simulink model "test_velocity_control_2"  (R2015a)
settings: Solver=FixedStepDiscrete  StartTime=0.0  StopTime=inf  FixedStep=sample_time  RelTol=1e-3
undefined symbols (not defined in the file or in its folder): A_lpf_fourbar_angles, A_lpf_imu, A_lpf_lateral_angle, B1_lpf_fourbar_angles, B1_lpf_imu, B1_lpf_lateral_angle, B2_lpf_fourbar_angles, B2_lpf_imu, B2_lpf_lateral_angle, control_start_time, kp_velocity_swing_trajectory, sample_time, swing_test_frequency, swing_test_leg_angle_amplitude, swing_test_leg_angle_bias, swing_test_leg_length_amplitude, swing_test_leg_length_bias, swing_test_length_angle_phase, swing_test_right_left_phase
libraries: simulink x6
settings Model: CovSFcnEnable=off  Creator=wmartin  LastModifiedBy=wmartin
settings SolverCC: EnableConcurrentExecution=on
settings DataIOCC: LimitDataPoints=off  MaxDataPoints=1000000000  SaveFormat=StructureWithTime  SignalLogging=off  DSMLogging=off  VisualizeSimOutput=off
settings OptimizationCC: BlockReduction=off  OptimizeBlockIOStorage=off  BufferReuse=off  GlobalBufferReuse=off  ExpressionFolding=off  ExpressionDepthLimit=2147483647  LocalBlockOutputs=off  SimCompilerOptimization=on
settings DebuggingCC: UnderspecifiedInitializationDetection=Classic  MergeDetectMultiDrivingBlocksExec=none  SolverPrmCheckMsg=warning  StateNameClashWarn=warning
settings HardwareCC: ProdIntDivRoundTo=Zero  ProdEndianess=LittleEndian  ProdLongLongMode=on  ProdHWDeviceType=Generic->32-bit x86 compatible
settings ModelReferenceCC: UpdateModelReferenceTargets=IfOutOfDate  ModelReferenceNumInstancesAllowed=Single  ModelReferenceMinAlgLoopOccurrences=on
settings RTWCC: SystemTargetFile=slrt.tlc  TemplateMakefile=slrt_default_tmf  Description=Simulink Real-Time  RTWVerbose=off  RTWCompilerOptimization=on
settings CodeAppCC: MaxIdLength=256
settings SimulinkRealTimeCC: GeneratePreprocessorConditionals=Disable all  RL32LogBufSizeModifier=1e8

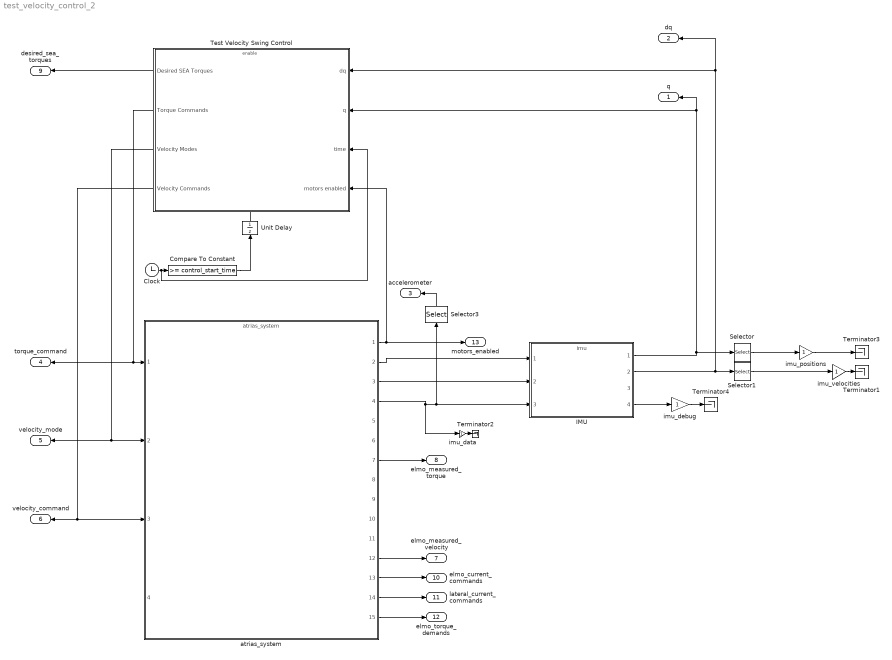
== system test_velocity_control_2 ==
  Clock : Clock
  Compare To Constant : simulink/Logic and Bit Operations/Compare To Constant  relop=>=  const=control_start_time  OutDataTypeStr=boolean
  IMU : ModelReference  ModelNameDialog=imu  SimulationMode=Normal  ModelReferenceVersion=1.2455  CopyOfModelName=imu  DefaultDataLogging=on
  Selector : Selector  InputPortWidth=13  Indices=[11 12 13]
  Selector1 : Selector  InputPortWidth=13  Indices=[11 12 13]
  Selector3 : Selector  InputPortWidth=9  Indices=[4 5 6]
  Terminator{1..4} (4 alike) : Terminator
  Test Velocity Swing Control : Subsystem
  Unit Delay : UnitDelay  SampleTime=-1
  atrias_system : ModelReference  ModelNameDialog=atrias_system  SimulationMode=Normal  ModelReferenceVersion=1.2965  CopyOfModelName=atrias_system  DefaultDataLogging=on
  imu_data : Gain
  imu_debug : Gain
  imu_positions : Gain
  imu_velocities : Gain
  q : Outport
  dq : Outport  Port=2
  accelerometer : Outport  Port=3  SampleTime=sample_time
  torque_command : Outport  Port=4  SampleTime=sample_time
  velocity_mode : Outport  Port=5  SampleTime=sample_time
  velocity_command : Outport  Port=6  SampleTime=sample_time
  elmo_measured_velocity : Outport  Port=7  SampleTime=sample_time
  elmo_measured_torque : Outport  Port=8  SampleTime=sample_time
  desired_sea_torques : Outport  Port=9  SampleTime=sample_time
  elmo_current_commands : Outport  Port=10  SampleTime=sample_time
  lateral_current_commands : Outport  Port=11  SampleTime=sample_time
  elmo_torque_demands : Outport  Port=12  SampleTime=sample_time
  motors_enabled : Outport  Port=13  SampleTime=sample_time
  wires:
  Clock/1 -> Test Velocity Swing Control/3(time), Compare To Constant/1
  imu_data/1 -> Terminator2/1
  imu_velocities/1 -> Terminator1/1
  imu_positions/1 -> Terminator3/1
  imu_debug/1 -> Terminator4/1
  IMU/4 -> imu_debug/1
  Selector/1 -> imu_positions/1
  Selector1/1 -> imu_velocities/1
  atrias_system/2 -> IMU/1
  IMU/1 -> q/1, Test Velocity Swing Control/2(q), Selector/1
  atrias_system/3 -> IMU/2
  atrias_system/4 -> imu_data/1, IMU/3, Selector3/1
  IMU/2 -> Selector1/1, dq/1, Test Velocity Swing Control/1(dq)
  Selector3/1 -> accelerometer/1
  atrias_system/7 -> elmo_measured_torque/1
  Test Velocity Swing Control/4(Velocity Commands) -> atrias_system/3, velocity_command/1
  Test Velocity Swing Control/3(Velocity Modes) -> atrias_system/2, velocity_mode/1
  Test Velocity Swing Control/2(Torque Commands) -> torque_command/1, atrias_system/1
  Test Velocity Swing Control/1(Desired SEA Torques) -> desired_sea_torques/1
  Unit Delay/1 -> Test Velocity Swing Control/Enable
  Compare To Constant/1 -> Unit Delay/1
  atrias_system/15 -> elmo_torque_demands/1
  atrias_system/14 -> lateral_current_commands/1
  atrias_system/13 -> elmo_current_commands/1
  atrias_system/12 -> elmo_measured_velocity/1
  atrias_system/1 -> Test Velocity Swing Control/4(motors enabled), motors_enabled/1

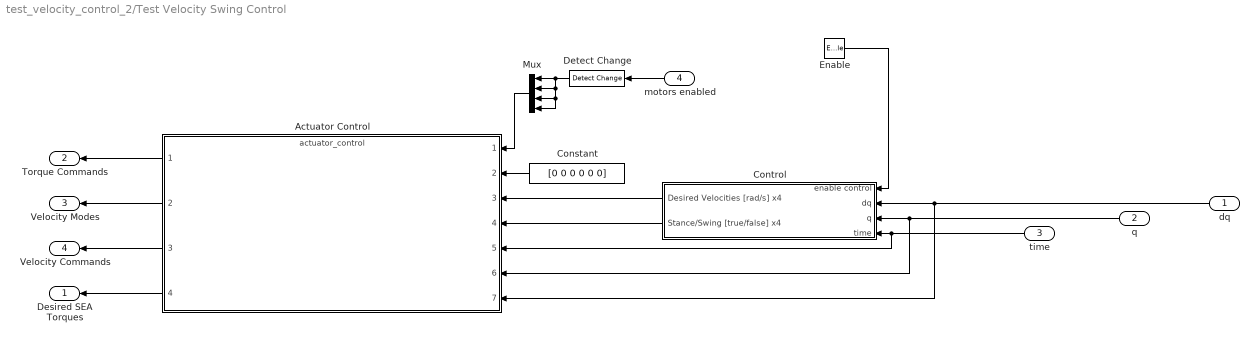
== system test_velocity_control_2/Test Velocity Swing Control ==
  dq : Inport
  q : Inport  Port=2
  time : Inport  Port=3
  motors enabled : Inport  Port=4
  Enable : EnablePort  StatesWhenEnabling=reset  PropagateVarSize=During execution  ShowOutputPort=on
  Actuator Control : ModelReference  ModelNameDialog=actuator_control  SimulationMode=Normal  ModelReferenceVersion=1.1228  CopyOfModelName=actuator_control  DefaultDataLogging=on
  Constant : Constant  Value=[0 0 0 0 0 0]
  Control : Subsystem
  Detect Change : simulink/Logic and Bit Operations/Detect Change  vinit=0  InputProcessing=Inherited  OutDataTypeStr=boolean
  Mux : Mux
  Desired SEA Torques : Outport
  Torque Commands : Outport  Port=2
  Velocity Modes : Outport  Port=3
  Velocity Commands : Outport  Port=4
  wires:
  Control/1(Desired Velocities [rad/s] x4) -> Actuator Control/3
  dq/1 -> Actuator Control/7, Control/2(dq)
  q/1 -> Actuator Control/6, Control/3(q)
  Actuator Control/3 -> Velocity Commands/1
  Actuator Control/2 -> Velocity Modes/1
  Actuator Control/1 -> Torque Commands/1
  time/1 -> Actuator Control/5, Control/4(time)
  Actuator Control/4 -> Desired SEA Torques/1
  motors enabled/1 -> Detect Change/1
  Control/2(Stance/Swing [true/false] x4) -> Actuator Control/4
  Mux/1 -> Actuator Control/1
  Detect Change/1 -> Mux/4, Mux/3, Mux/2, Mux/1
  Enable/1 -> Control/1(enable control)
  Constant/1 -> Actuator Control/2

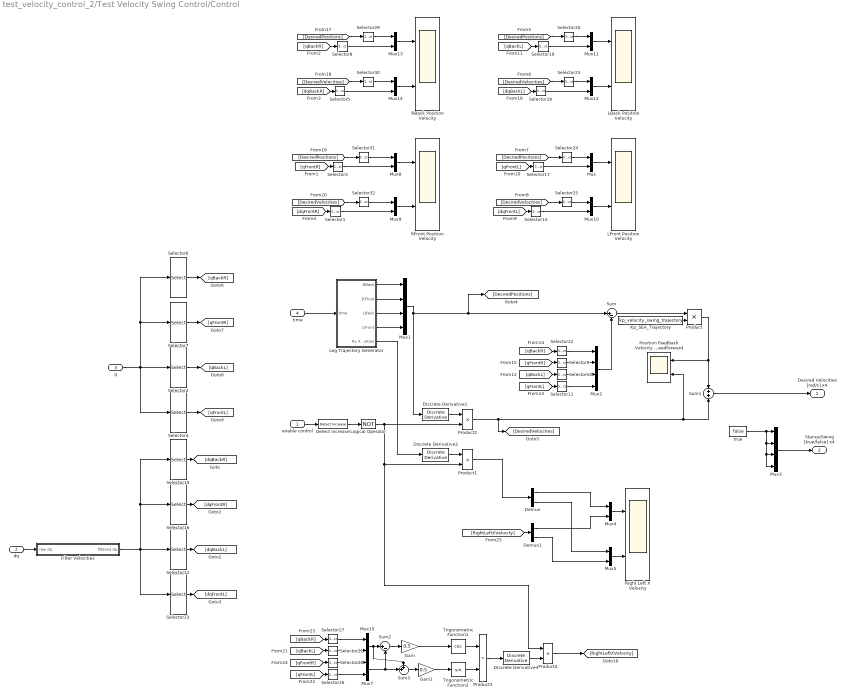
== system test_velocity_control_2/Test Velocity Swing Control/Control ==
  enable control : Inport
  dq : Inport  Port=2
  q : Inport  Port=3
  time : Inport  Port=4
  Demux : Demux  Outputs=2
  Demux1 : Demux  Outputs=2
  Detect Increase : simulink/Logic and Bit Operations/Detect Increase  vinit=0.0  InputProcessing=Inherited  OutDataTypeStr=boolean
  Discrete Derivative1 : simulink/Discrete/Discrete Derivative  gainval=1.0  ICPrevScaledInput=0.0  OutMin=[]  OutMax=[]  OutDataType=fixdt(1, 16)  OutScaling=2^-10  DoSatur=off
  Discrete Derivative2 : simulink/Discrete/Discrete Derivative  gainval=1.0  ICPrevScaledInput=0.0  OutMin=[]  OutMax=[]  OutDataType=fixdt(1, 16)  OutScaling=2^-10  DoSatur=off
  Discrete Derivative3 : simulink/Discrete/Discrete Derivative  gainval=1.0  ICPrevScaledInput=0.0  OutMin=[]  OutMax=[]  OutDataType=fixdt(1, 16)  OutScaling=2^-10  DoSatur=off
  Filter Velocities : Subsystem
  Gain : Gain  Gain=0.5
  Gain1 : Gain  Gain=0.5
  Kp_SEA_Trajectory : Constant  Value=kp_velocity_swing_trajectory
  LBack Position Velocity : Scope  NumInputPorts=2
      settings: YMin=2.175~-0.275  YMax=2.55~0.275  SampleInput=on
  LFront Position Velocity : Scope  NumInputPorts=2
      settings: YMin=2.175~-0.275  YMax=2.55~0.275  SaveName=ScopeData4  SampleInput=on
  Leg Trajectory Generator : Subsystem
  Logical Operator : Logic  Operator=NOT  AllPortsSameDT=off  OutDataTypeStr=boolean
  Mux{,4..5,7..15} (12 alike) : Mux  Inputs=2
  Mux1 : Mux
  Mux2 : Mux
  Mux3 : Mux
  Position Feedback Velocity Feedforward : Scope  NumInputPorts=2
      settings: YMin=-4~-0.9  YMax=4.5~1  SaveName=ScopeData7  SampleInput=on
  Product{,1..4} (5 alike) : Product
  RBack Position Velocity : Scope  NumInputPorts=2
      settings: YMin=3.75~-2.25  YMax=4.125~2.25  SampleInput=on
  RFront Position Velocity : Scope  NumInputPorts=2
      settings: YMin=2.175~-0.275  YMax=2.55~0.275  SaveName=ScopeData2  SampleInput=on
  Right Left X Velocity : Scope  NumInputPorts=2
      settings: YMin=-130~-10  YMax=10~65  SaveName=ScopeData3  SampleInput=on
  Selector{1,3,5,8..11,14,17..19,21..22,26..28} (16 alike) : Selector  InputPortWidth=2  Indices=[2]
  Selector12 : Selector  InputPortWidth=13  Indices=[5 6]
  Selector13 : Selector  InputPortWidth=13  Indices=[7 8]
  Selector15 : Selector  InputPortWidth=13  Indices=[1 2]
  Selector16 : Selector  InputPortWidth=13  Indices=[3 4]
  Selector2 : Selector  InputPortWidth=13  Indices=[5 6]
  Selector20 : Selector  InputPortWidth=4  Indices=[3]
  Selector23 : Selector  InputPortWidth=4  Indices=[3]
  Selector24 : Selector  InputPortWidth=4  Indices=[4]
  Selector25 : Selector  InputPortWidth=4  Indices=[4]
  Selector29 : Selector  InputPortWidth=4  Indices=[1]
  Selector30 : Selector  InputPortWidth=4  Indices=[1]
  Selector31 : Selector  InputPortWidth=4  Indices=[2]
  Selector32 : Selector  InputPortWidth=4  Indices=[2]
  Selector4 : Selector  InputPortWidth=13  Indices=[7 8]
  Selector6 : Selector  InputPortWidth=13  Indices=[1 2]
  Selector7 : Selector  InputPortWidth=13  Indices=[3 4]
  Sum : Sum  Inputs=|+-
  Sum1 : Sum  Inputs=+|+
  Sum2 : Sum  Inputs=|+-
  Sum3 : Sum  Inputs=++|
  Trigonometric Function1 : Trigonometry  Operator=cos
  Trigonometric Function2 : Trigonometry
  true : Constant  Value=false
  Desired Velocities [rad/s] x4 : Outport  InitialOutput=[0 0 0 0 0 0]
  Stance/Swing [true/false] x4 : Outport  Port=2  InitialOutput=[false false false false]
  wires:
  dq/1 -> Filter Velocities/1(raw dq)
  Filter Velocities/1(filtered dq) -> Selector12/1, Selector16/1, Selector15/1, Selector13/1
  Selector15/1 -> [dqBackR]
  Selector16/1 -> [dqFrontR]
  Selector12/1 -> [dqBackL]
  Selector13/1 -> [dqFrontL]
  Selector6/1 -> [qBackR]
  Selector7/1 -> [qFrontR]
  Selector2/1 -> [qBackL]
  Selector4/1 -> [qFrontL]
  q/1 -> Selector4/1, Selector6/1, Selector7/1, Selector2/1
  Mux2/1 -> Sum/2
  [qBackR] -> Selector22/1
  Selector22/1 -> Mux2/1
  Selector10/1 -> Mux2/3
  Selector9/1 -> Mux2/2
  Selector11/1 -> Mux2/4
  [qFrontR] -> Selector9/1
  [qBackL] -> Selector10/1
  [qFrontL] -> Selector11/1
  Mux1/1 -> Discrete Derivative1/1, [DesiredPositions], Sum/1
  Sum/1 -> Product/1
  Product/1 -> Position Feedback Velocity Feedforward/1, Sum1/1
  Sum1/1 -> Desired Velocities [rad/s] x4/1
  Product2/1 -> [DesiredVelocities], Sum1/2, Position Feedback Velocity Feedforward/2
  Mux/1 -> LFront Position Velocity/1
  Mux10/1 -> LFront Position Velocity/2
  [dqFrontL] -> Selector14/1
  Selector14/1 -> Mux10/2
  [qFrontL] -> Selector17/1
  Selector17/1 -> Mux/2
  Kp_SEA_Trajectory/1 -> Product/2
  true/1 -> Mux3/4, Mux3/3, Mux3/2, Mux3/1
  Mux3/1 -> Stance/Swing [true/false] x4/1
  Mux11/1 -> LBack Position Velocity/1
  Mux12/1 -> LBack Position Velocity/2
  [qBackL] -> Selector19/1
  Selector19/1 -> Mux11/2
  [dqBackL] -> Selector18/1
  Selector18/1 -> Mux12/2
  Leg Trajectory Generator/3(LBack) -> Mux1/3
  Leg Trajectory Generator/4(LFront) -> Mux1/4
  Leg Trajectory Generator/1(RBack) -> Mux1/1
  Mux14/1 -> RBack Position Velocity/2
  Mux13/1 -> RBack Position Velocity/1
  Mux9/1 -> RFront Position Velocity/2
  Mux8/1 -> RFront Position Velocity/1
  [dqBackR] -> Selector5/1
  [qBackR] -> Selector8/1
  [qFrontR] -> Selector3/1
  [dqFrontR] -> Selector1/1
  Selector1/1 -> Mux9/2
  Selector3/1 -> Mux8/2
  Selector8/1 -> Mux13/2
  Selector5/1 -> Mux14/2
  Leg Trajectory Generator/2(RFront) -> Mux1/2
  enable control/1 -> Detect Increase/1
  Detect Increase/1 -> Logical Operator/1
  Discrete Derivative1/1 -> Product2/1
  [DesiredPositions] -> Selector20/1
  Selector20/1 -> Mux11/1
  [DesiredVelocities] -> Selector23/1
  Selector23/1 -> Mux12/1
  [DesiredPositions] -> Selector24/1
  [DesiredVelocities] -> Selector25/1
  Selector25/1 -> Mux10/1
  Selector24/1 -> Mux/1
  [DesiredPositions] -> Selector29/1
  Selector29/1 -> Mux13/1
  [DesiredVelocities] -> Selector30/1
  Selector30/1 -> Mux14/1
  [DesiredPositions] -> Selector31/1
  [DesiredVelocities] -> Selector32/1
  Selector32/1 -> Mux9/1
  Selector31/1 -> Mux8/1
  time/1 -> Leg Trajectory Generator/1(time)
  Trigonometric Function1/1 -> Product3/1
  Trigonometric Function2/1 -> Product3/2
  [qFrontL] -> Selector26/1
  [qBackL] -> Selector21/1
  [qFrontR] -> Selector28/1
  Selector26/1 -> Mux7/2
  Selector28/1 -> Mux7/1
  Selector21/1 -> Mux15/2
  Selector27/1 -> Mux15/1
  [qBackR] -> Selector27/1
  Mux15/1 -> Sum2/1, Sum3/1
  Mux7/1 -> Sum2/2, Sum3/2
  Sum2/1 -> Gain/1
  Gain/1 -> Trigonometric Function1/1
  Sum3/1 -> Gain1/1
  Gain1/1 -> Trigonometric Function2/1
  Product3/1 -> Discrete Derivative3/1
  Discrete Derivative3/1 -> Product4/2
  Logical Operator/1 -> Product1/2, Product4/1, Product2/2
  Discrete Derivative2/1 -> Product1/1
  Leg Trajectory Generator/5(RL X Position) -> Discrete Derivative2/1
  Demux/1 -> Mux4/1
  Demux/2 -> Mux5/1
  Mux4/1 -> Right Left X Velocity/1
  Mux5/1 -> Right Left X Velocity/2
  [RightLeftXVelocity] -> Demux1/1
  Demux1/1 -> Mux4/2
  Demux1/2 -> Mux5/2
  Product1/1 -> Demux/1
  Product4/1 -> [RightLeftXVelocity]

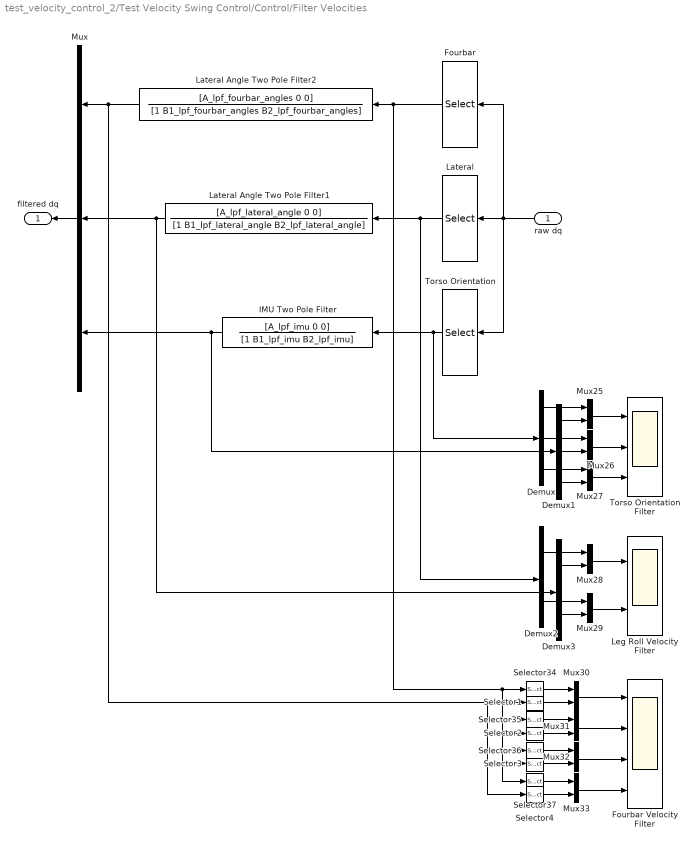
== system test_velocity_control_2/Test Velocity Swing Control/Control/Filter Velocities ==
  raw dq : Inport
  Demux : Demux  Outputs=3
  Demux1 : Demux  Outputs=3
  Demux2 : Demux  Outputs=2
  Demux3 : Demux  Outputs=2
  Fourbar : Selector  InputPortWidth=13  Indices=[1 2 3 4 5 6 7 8]
  Fourbar Velocity Filter : Scope  NumInputPorts=4
      settings: YMin=-0.55~-0.4~-0.4~-0.6  YMax=0.25~0.7~0.45~0.5  SaveName=ScopeData14  SampleInput=on
  IMU Two Pole Filter : DiscreteTransferFcn  Numerator=[A_lpf_imu 0 0]  Denominator=[1 B1_lpf_imu B2_lpf_imu]  SampleTime=sample_time
  Lateral : Selector  InputPortWidth=13  Indices=[9 10]
  Lateral Angle Two Pole Filter1 : DiscreteTransferFcn  Numerator=[A_lpf_lateral_angle 0 0]  Denominator=[1 B1_lpf_lateral_angle B2_lpf_lateral_angle]  SampleTime=sample_time
  Lateral Angle Two Pole Filter2 : DiscreteTransferFcn  Numerator=[A_lpf_fourbar_angles 0 0]  Denominator=[1 B1_lpf_fourbar_angles B2_lpf_fourbar_angles]  SampleTime=sample_time
  Leg Roll Velocity Filter : Scope  NumInputPorts=2
      settings: YMin=-0.225~-1.5  YMax=0.175~2.25  SaveName=LegRollFilter  SampleInput=on
  Mux : Mux  Inputs=3
  Mux{25..33} (9 alike) : Mux  Inputs=2
  Selector1 : Selector  InputPortWidth=8  Indices=[1 2]
  Selector2 : Selector  InputPortWidth=8  Indices=[3 4]
  Selector3 : Selector  InputPortWidth=8  Indices=[5 6]
  Selector34 : Selector  InputPortWidth=8  Indices=[1 2]
  Selector35 : Selector  InputPortWidth=8  Indices=[3 4]
  Selector36 : Selector  InputPortWidth=8  Indices=[5 6]
  Selector37 : Selector  InputPortWidth=8  Indices=[7 8]
  Selector4 : Selector  InputPortWidth=8  Indices=[7 8]
  Torso Orientation : Selector  InputPortWidth=13  Indices=[11 12 13]
  Torso Orientation Filter : Scope  NumInputPorts=3
      settings: YMin=-0.2~-0.03~-0.15  YMax=0.125~0.0275~0.15  SaveName=ScopeData13  SampleInput=on
  filtered dq : Outport
  wires:
  Lateral Angle Two Pole Filter2/1 -> Selector4/1, Selector3/1, Selector2/1, Selector1/1, Mux/1
  IMU Two Pole Filter/1 -> Demux1/1, Mux/3
  Mux/1 -> filtered dq/1
  raw dq/1 -> Fourbar/1, Torso Orientation/1, Lateral/1
  Lateral/1 -> Demux2/1, Lateral Angle Two Pole Filter1/1
  Torso Orientation/1 -> IMU Two Pole Filter/1, Demux/1
  Lateral Angle Two Pole Filter1/1 -> Demux3/1, Mux/2
  Mux25/1 -> Torso Orientation Filter/1
  Mux27/1 -> Torso Orientation Filter/3
  Mux26/1 -> Torso Orientation Filter/2
  Mux30/1 -> Fourbar Velocity Filter/1
  Mux32/1 -> Fourbar Velocity Filter/3
  Mux31/1 -> Fourbar Velocity Filter/2
  Mux33/1 -> Fourbar Velocity Filter/4
  Selector34/1 -> Mux30/1
  Fourbar/1 -> Selector34/1, Selector35/1, Selector36/1, Selector37/1, Lateral Angle Two Pole Filter2/1
  Selector35/1 -> Mux31/1
  Selector36/1 -> Mux32/1
  Selector37/1 -> Mux33/1
  Mux28/1 -> Leg Roll Velocity Filter/1
  Mux29/1 -> Leg Roll Velocity Filter/2
  Demux/1 -> Mux25/1
  Demux/2 -> Mux26/1
  Demux/3 -> Mux27/1
  Demux1/1 -> Mux25/2
  Demux1/2 -> Mux26/2
  Demux1/3 -> Mux27/2
  Demux2/2 -> Mux29/1
  Demux2/1 -> Mux28/1
  Demux3/1 -> Mux28/2
  Demux3/2 -> Mux29/2
  Selector4/1 -> Mux33/2
  Selector3/1 -> Mux32/2
  Selector2/1 -> Mux31/2
  Selector1/1 -> Mux30/2

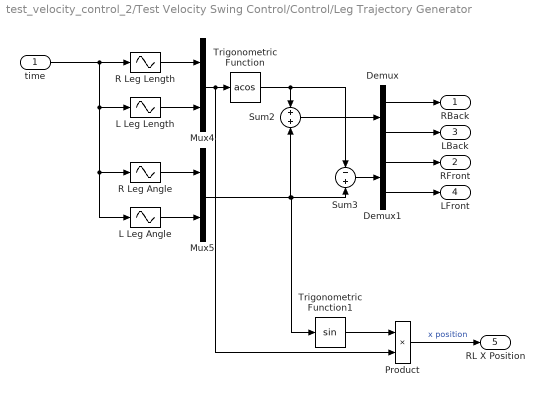
== system test_velocity_control_2/Test Velocity Swing Control/Control/Leg Trajectory Generator ==
  time : Inport
  Demux : Demux  Outputs=2
  Demux1 : Demux  Outputs=2
  L Leg Angle : Sin  TimeSource=Use external signal  Amplitude=swing_test_leg_angle_amplitude  Bias=swing_test_leg_angle_bias  Frequency=swing_test_frequency  Phase=swing_test_right_left_phase  SampleTime=0
  L Leg Length : Sin  TimeSource=Use external signal  Amplitude=swing_test_leg_length_amplitude  Bias=swing_test_leg_length_bias  Frequency=swing_test_frequency  Phase=swing_test_right_left_phase+swing_test_length_angle_phase  SampleTime=0
  Mux4 : Mux  Inputs=2
  Mux5 : Mux  Inputs=2
  Product : Product
  R Leg Angle : Sin  TimeSource=Use external signal  Amplitude=swing_test_leg_angle_amplitude  Bias=swing_test_leg_angle_bias  Frequency=swing_test_frequency  SampleTime=0
  R Leg Length : Sin  TimeSource=Use external signal  Amplitude=swing_test_leg_length_amplitude  Bias=swing_test_leg_length_bias  Frequency=swing_test_frequency  Phase=swing_test_length_angle_phase  SampleTime=0
  Sum2 : Sum  Inputs=+|+
  Sum3 : Sum  Inputs=-|+
  Trigonometric Function : Trigonometry  Operator=acos
  Trigonometric Function1 : Trigonometry
  RBack : Outport
  RFront : Outport  Port=2
  LBack : Outport  Port=3
  LFront : Outport  Port=4
  RL X Position : Outport  Port=5
  wires:
  Product/1 -> RL X Position/1  "x position"
  Trigonometric Function1/1 -> Product/1
  Demux1/1 -> RFront/1
  Demux/1 -> RBack/1
  Demux1/2 -> LFront/1
  Demux/2 -> LBack/1
  R Leg Angle/1 -> Mux5/1
  time/1 -> L Leg Angle/1, R Leg Angle/1, L Leg Length/1, R Leg Length/1
  Sum3/1 -> Demux1/1
  L Leg Angle/1 -> Mux5/2
  R Leg Length/1 -> Mux4/1
  L Leg Length/1 -> Mux4/2
  Mux5/1 -> Sum2/2, Sum3/2, Trigonometric Function1/1
  Sum2/1 -> Demux/1
  Mux4/1 -> Trigonometric Function/1, Product/2
  Trigonometric Function/1 -> Sum2/1, Sum3/1
